simulink model "Simulink_Model"  (R2020b)
settings: Solver=FixedStepAuto  StartTime=0.0  StopTime=12  FixedStep=1  RelTol=1e-3
values from neighbouring files (symbols this model uses):
  ConstantA = Constants{1}    [Load_config.m]
  ConstantB = Constants{2}    [Load_config.m]
  ConstantC = Constants{3}    [Load_config.m]
  ConstantD = Constants{4}    [Load_config.m]
  ConstantE = Constants{5}    [Load_config.m]
  ConstantF = Constants{6}    [Load_config.m]
  ConstantG = Constants{7}    [Load_config.m]
  ConstantH = Constants{8}    [Load_config.m]
  ConstantI = Constants{9}    [Load_config.m]
  ConstantJ = Constants{18}    [Load_config.m]
  ConstantK = Constants{19}    [Load_config.m]
  ConstantL = Constants{20}    [Load_config.m]
  ConstantM = Constants{21}    [Load_config.m]
  ConstantO = Constants{22}    [Load_config.m]
undefined symbols (not defined in the file or in its folder): A1052, A2, F2, G1052, H2, K1052
libraries: simulink x32, sldvlib x22
(part 1 of 3)
settings Model: Creator=Marcus  LastModifiedBy=marcushanikat
settings ConfigComp: DVMode=PropertyProving  DVMaxProcessTime=36000  DVParameters=on  DVParametersUseConfig=on  DVTestConditions=EnableAll  DVTestObjectives=EnableAll  DVMaxTestCaseSteps=1000  DVTestSuiteOptimization=LongTestcases  DVDetectOutOfBounds=on  DVMaxViolationSteps=8

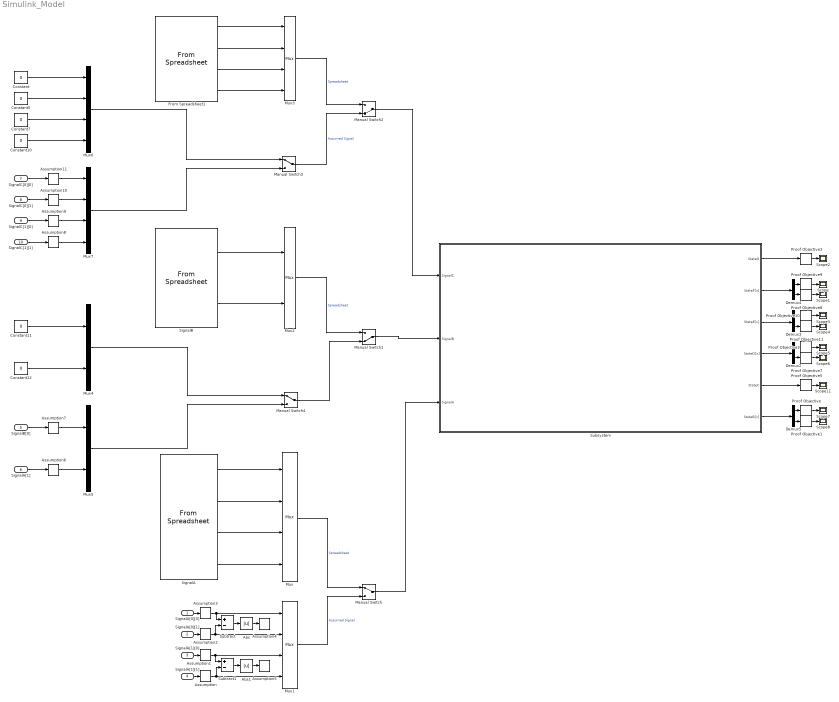
== system Simulink_Model ==
  SignalA[0][0] : Inport  OutDataTypeStr=int32
  SignalA[0][1] : Inport  Port=2  OutDataTypeStr=int32
  SignalA[1][0] : Inport  Port=3  OutDataTypeStr=int32
  SignalA[1][1] : Inport  Port=4  OutDataTypeStr=int32
  SignalB[0] : Inport  Port=5
  SignalA[1] : Inport  Port=6
  SignalC[0][0] : Inport  Port=7
  SignalC[0][1] : Inport  Port=8
  SignalC[1][0] : Inport  Port=9
  SignalC[1][1] : Inport  Port=10
  Abs : Abs
  Abs1 : Abs
  Assumption{,1..3} (4 alike) : sldvlib/Objectives and Constraints/Assumption  enabled=on  customAVTBlockType=Assumption  intervals={0 1 2 3 4 5}  initial=off  dispValues=off  outEnabled=on
      settings: SourceProductBaseCode=SL
  Assumption{8..11} (4 alike) : sldvlib/Objectives and Constraints/Assumption  enabled=on  customAVTBlockType=Assumption  intervals={0 1}  initial=off  dispValues=off  outEnabled=on
      settings: SourceProductBaseCode=SL
  Assumption4 : sldvlib/Objectives and Constraints/Assumption  enabled=on  customAVTBlockType=Assumption  intervals={0 1}  initial=off  dispValues=off  outEnabled=off
      settings: SourceProductBaseCode=SL
  Assumption5 : sldvlib/Objectives and Constraints/Assumption  enabled=on  customAVTBlockType=Assumption  intervals={0 1}  initial=off  dispValues=off  outEnabled=off
      settings: SourceProductBaseCode=SL
  Assumption6 : sldvlib/Objectives and Constraints/Assumption  enabled=on  customAVTBlockType=Assumption  intervals={0 1 2}  initial=off  dispValues=off  outEnabled=on
      settings: SourceProductBaseCode=SL
  Assumption7 : sldvlib/Objectives and Constraints/Assumption  enabled=on  customAVTBlockType=Assumption  intervals={0 1 2}  initial=off  dispValues=off  outEnabled=on
      settings: SourceProductBaseCode=SL
  Constant{,5,7,10..12} (6 alike) : Constant  Value=0
  Demux{2..5} (4 alike) : Demux  Outputs=2
  From Spreadsheet1 : FromSpreadsheet  FileName=/Users/marcushanikat/Documents/git/Master_thesis/Excel/Signals.xlsx  SheetName=Signals  Range=A2:A1052,H2:K1052  OutDataTypeStr=int32
  Manual Switch : ManualSwitch
  Manual Switch1 : ManualSwitch  CurrentSetting=0
  Manual Switch2 : ManualSwitch  CurrentSetting=0
  Manual Switch3 : ManualSwitch
  Manual Switch4 : ManualSwitch
  Mux{,1,3,6..7} (5 alike) : Mux
  Mux2 : Mux  Inputs=2
  Mux4 : Mux  Inputs=2
  Mux5 : Mux  Inputs=2
  Proof Objective{,1..3,5,7..11} (10 alike) : sldvlib/Objectives and Constraints/Proof Objective  enabled=off  customAVTBlockType=Proof Objective  intervals={0}  dispValues=off  outEnabled=on  enableStopSim=off
      settings: SourceProductBaseCode=SL
  Scope{,1..8,11} (10 alike) : Scope
  SignalA : FromSpreadsheet  FileName=/Users/marcushanikat/Documents/git/Master_thesis/Excel/Signals.xlsx  SheetName=Signals  Range=A2:E1052  OutDataTypeStr=int32
  SignalB : FromSpreadsheet  FileName=/Users/marcushanikat/Documents/git/Master_thesis/Excel/Signals.xlsx  SheetName=Signals  Range=A2:A1052,F2:G1052  OutDataTypeStr=int32
  Subsystem : Subsystem
  Subtract : Sum  Inputs=+-
  Subtract1 : Sum  Inputs=+-
  wires:
  SignalA[1][0]/1 -> Assumption1/1
  SignalA[1][1]/1 -> Assumption/1
  Assumption/1 -> Subtract1/2, Mux1/4
  SignalA/3 -> Mux/3
  SignalA/4 -> Mux/4
  SignalA/1 -> Mux/1
  SignalA/2 -> Mux/2
  Assumption1/1 -> Subtract1/1, Mux1/3
  Manual Switch/1 -> Subsystem/3(SignalA)
  Mux1/1 -> Manual Switch/2  "Assumed Signal"
  Mux/1 -> Manual Switch/1  "Spreadsheet"
  SignalB/2 -> Mux2/2
  SignalB/1 -> Mux2/1
  From Spreadsheet1/1 -> Mux3/1
  From Spreadsheet1/2 -> Mux3/2
  From Spreadsheet1/3 -> Mux3/3
  From Spreadsheet1/4 -> Mux3/4
  SignalA[1]/1 -> Assumption6/1
  SignalB[0]/1 -> Assumption7/1
  SignalC[1][1]/1 -> Assumption8/1
  SignalC[0][1]/1 -> Assumption10/1
  SignalC[0][0]/1 -> Assumption11/1
  SignalC[1][0]/1 -> Assumption9/1
  Manual Switch1/1 -> Subsystem/2(SignalB)
  Mux2/1 -> Manual Switch1/1  "Spreadsheet"
  Manual Switch2/1 -> Subsystem/1(SignalC)
  Manual Switch3/1 -> Manual Switch2/2  "Assumed Signal"
  Mux3/1 -> Manual Switch2/1  "Spreadsheet"
  Subsystem/6(StateB[x]) -> Demux5/1
  Subsystem/3(StateE[x]) -> Demux3/1
  Subsystem/2(StateF[x]) -> Demux4/1
  Subsystem/4(StateD[x]) -> Demux2/1
  Subsystem/5(StateC) -> Proof Objective5/1
  Demux5/1 -> Proof Objective/1
  Proof Objective/1 -> Scope7/1
  Demux5/2 -> Proof Objective1/1
  Proof Objective1/1 -> Scope8/1
  Demux2/1 -> Proof Objective2/1
  Proof Objective2/1 -> Scope5/1
  Proof Objective3/1 -> Scope2/1
  Subsystem/1(StateG) -> Proof Objective3/1
  Proof Objective5/1 -> Scope11/1
  Subtract/1 -> Abs/1
  Assumption3/1 -> Subtract/1, Mux1/1
  Assumption2/1 -> Subtract/2, Mux1/2
  SignalA[0][1]/1 -> Assumption2/1
  SignalA[0][0]/1 -> Assumption3/1
  Abs/1 -> Assumption4/1
  Subtract1/1 -> Abs1/1
  Abs1/1 -> Assumption5/1
  Constant10/1 -> Mux6/4
  Constant7/1 -> Mux6/3
  Constant5/1 -> Mux6/2
  Constant/1 -> Mux6/1
  Assumption11/1 -> Mux7/1
  Assumption10/1 -> Mux7/2
  Assumption9/1 -> Mux7/3
  Assumption8/1 -> Mux7/4
  Mux7/1 -> Manual Switch3/2
  Mux6/1 -> Manual Switch3/1
  Constant11/1 -> Mux4/1
  Constant12/1 -> Mux4/2
  Assumption7/1 -> Mux5/1
  Assumption6/1 -> Mux5/2
  Manual Switch4/1 -> Manual Switch1/2
  Mux5/1 -> Manual Switch4/2
  Mux4/1 -> Manual Switch4/1
  Demux2/2 -> Proof Objective7/1
  Proof Objective7/1 -> Scope6/1
  Demux4/2 -> Proof Objective8/1
  Proof Objective8/1 -> Scope1/1
  Demux4/1 -> Proof Objective9/1
  Proof Objective9/1 -> Scope/1
  Demux3/1 -> Proof Objective10/1
  Proof Objective10/1 -> Scope3/1
  Demux3/2 -> Proof Objective11/1
  Proof Objective11/1 -> Scope4/1

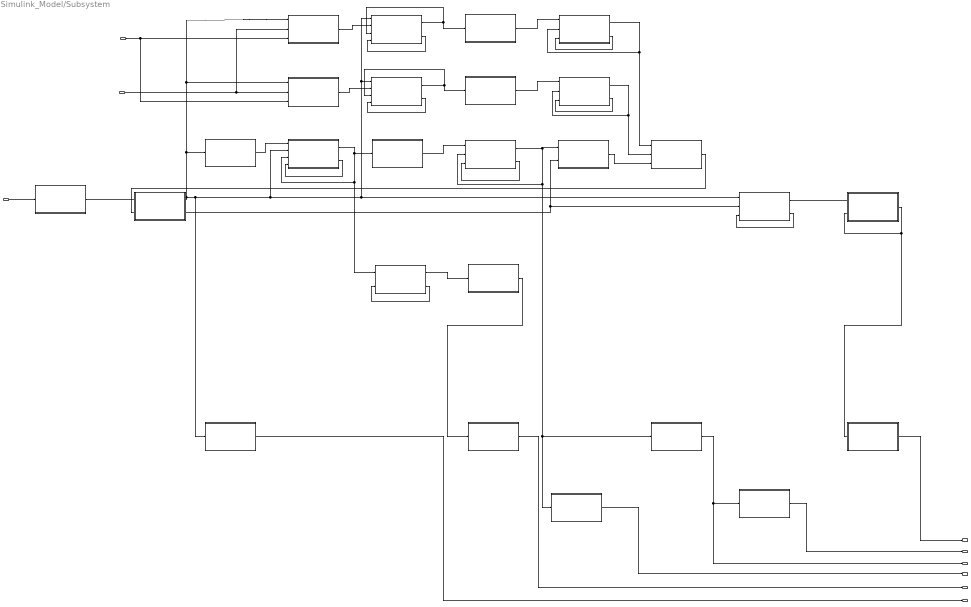
== system Simulink_Model/Subsystem ==
  SignalC : Inport
  SignalB : Inport  Port=2
  SignalA : Inport  Port=3
  Requirement1 : Subsystem  TreatAsAtomicUnit=on
  Requirement10 : Subsystem  TreatAsAtomicUnit=on
  Requirement11 : Subsystem  TreatAsAtomicUnit=on
  Requirement12 : Subsystem  TreatAsAtomicUnit=on
  Requirement14 : Subsystem  TreatAsAtomicUnit=on
  Requirement15 : Subsystem  TreatAsAtomicUnit=on
  Requirement2 : Subsystem  TreatAsAtomicUnit=on
  Requirement20 : Subsystem  TreatAsAtomicUnit=on
  Requirement21 : Subsystem  TreatAsAtomicUnit=on
  Requirement23 : Subsystem  TreatAsAtomicUnit=on
  Requirement24 : Subsystem  TreatAsAtomicUnit=on
  Requirement25 : Subsystem  TreatAsAtomicUnit=on
  Requirement26 : Subsystem  TreatAsAtomicUnit=on
  Requirement3 : Subsystem  TreatAsAtomicUnit=on
  Requirement4 : Subsystem  TreatAsAtomicUnit=on
  Requirement5 : Subsystem  TreatAsAtomicUnit=on
  Requirement6 : Subsystem  TreatAsAtomicUnit=on
  Requirement7 : Subsystem  TreatAsAtomicUnit=on
  Requirement8 : Subsystem  TreatAsAtomicUnit=on
  Requirement9 : Subsystem  TreatAsAtomicUnit=on
  Verification2 : Subsystem  TreatAsAtomicUnit=on
  Verification3 : Subsystem  TreatAsAtomicUnit=on
  Verification4 : Subsystem  TreatAsAtomicUnit=on
  Verification5 : Subsystem  TreatAsAtomicUnit=on
  Verification6 : Subsystem  TreatAsAtomicUnit=on
  Verification8 : Subsystem  TreatAsAtomicUnit=on
  StateG : Outport
  StateF[x] : Outport  Port=2
  StateE[x] : Outport  Port=3
  StateD[x] : Outport  Port=4
  StateC : Outport  Port=5
  StateB[x] : Outport  Port=6
  wires:
  Requirement7/1(OutputJ) -> Requirement8/2(OutputJ)  "OutputJ"
  Requirement2/2(OutputC) -> Requirement20/2(OutputC), Requirement25/2(OutputC)  "OutputC"
  Requirement14/2(OutputS) -> Requirement14/3(OutputSOld)
  Requirement15/1(OutputT) -> Requirement21/1(OutputT), Requirement15/2(OutputTOld)  "OutputT"
  Requirement20/1(OutputV) -> Requirement21/3(OutputV)  "OutputV"
  Requirement2/1(OutputB) -> Verification2/1(OutputB), Requirement4/2(OutputB), Requirement25/1(OutputB), Requirement8/1(OutputB), Requirement6/1(OutputB), Requirement7/1(OutputB), Requirement5/1(OutputB), Requirement3/1(OutputB)  "OutputB"
  Requirement4/1(OutputE) -> Requirement4/3(OutputEOld), Requirement23/1(OutputE), Requirement9/1(OutputE)  "OutputE"
  Requirement12/1(OutputP) -> Requirement12/2(OutputPOld), Verification5/1(OutputP), Verification4/1(OutputP), Requirement20/1(OutputP)  "OutputP"
  Requirement10/1(OutputN) -> Requirement14/1(OutputN)  "OutputN"
  Requirement14/1(OutputR) -> Requirement14/2(OutputROld), Requirement21/2(OutputR)  "OutputR"
  Requirement21/1(OutputW) -> Requirement2/2(OutputW)
  Requirement24/1(OutputY) -> Verification3/1(OutputY)  "OutputY"
  Requirement15/2(OutputU) -> Requirement15/3(OutputUOld)
  Requirement11/1(OutputO) -> Requirement15/1(OutputO)  "OutputO"
  Verification8/1(StateG) -> StateG/1  "StateG"
  Verification3/1(StateC) -> StateC/1  "StateC"
  Requirement4/2(OutputF) -> Requirement4/4(OutputFOld)
  Verification5/1(StateE) -> Verification6/1(StateE), StateE[x]/1  "StateE"
  Requirement5/1(OutputG) -> Requirement6/2(OutputG)  "OutputG"
  Verification4/1(StateD) -> StateD[x]/1  "StateD"
  Requirement25/2(OutputAA) -> Requirement25/3(OutputAAOld)
  Requirement3/1(OutputD) -> Requirement4/1(OutputD)  "OutputD"
  Requirement25/1(OutputZ) -> Requirement26/1(OutputZ)  "OutputZ"
  Verification2/1(StateB) -> StateB[x]/1  "StateB"
  Requirement8/1(OutputK) -> Requirement11/1(OutputK), Requirement8/3(OutputKOld)  "OutputK"
  Verification6/1(StateF) -> StateF[x]/1  "StateF"
  Requirement6/1(OutputH) -> Requirement6/3(OutputHOld), Requirement10/1(OutputH)  "OutputH"
  Requirement8/2(OutputL) -> Requirement8/4(OutputLOld)
  Requirement23/2(OutputE(t-2)) -> Requirement23/2(OutputEOld)
  Requirement23/1(OutputX) -> Requirement24/1(OutputX)  "OutputX"
  SignalA/1 -> Requirement1/1(SignalA)
  Requirement1/1(OutputA) -> Requirement2/1(OutputA)
  Requirement12/2(OutputQ) -> Requirement12/3(OutputQOld)
  Requirement9/1(OutputM) -> Requirement12/1(OutputM)
  Requirement6/2(OutputI) -> Requirement6/4(OutputIOld)
  Requirement26/1(OutputAB) -> Verification8/1(OutputAB), Requirement26/2(OutputABOld)  "OutputAB"
  SignalC/1 -> Requirement5/3(SignalC), Requirement7/3(SignalC)
  SignalB/1 -> Requirement7/2(SignalB), Requirement5/2(SignalB)

== system Simulink_Model/Subsystem/Requirement1 ==
  note: Requirements implemented:
      | Requirement1
  SignalA : Inport
  Compare To Constant : simulink/Logic and Bit Operations/Compare To Constant  relop===  const=2  OutDataTypeStr=boolean
  Compare To Constant1 : simulink/Logic and Bit Operations/Compare To Constant  relop===  const=2  OutDataTypeStr=boolean
  Constant : Constant  Value=ConstantA
  Constant1 : Constant  Value=ConstantA
  Demux : Demux
  Gain{,1..3} (4 alike) : Gain  Gain=-1
  Mux : Mux
  Switch{,1..3} (4 alike) : Switch  Criteria=u2 > Threshold  OutDataTypeStr=int32
  OutputA : Outport
  wires:
  SignalA/1 -> Demux/1
  Constant1/1 -> Compare To Constant/1  "ConstantA"
  Compare To Constant/1 -> Switch1/2, Switch/2
  Demux/1 -> Gain/1, Switch/3
  Switch/1 -> Mux/1
  Gain/1 -> Switch/1
  Switch1/1 -> Mux/2
  Demux/2 -> Gain1/1, Switch1/3
  Gain1/1 -> Switch1/1
  Constant/1 -> Compare To Constant1/1  "ConstantA"
  Switch2/1 -> Mux/3
  Demux/3 -> Gain2/1, Switch2/3
  Gain2/1 -> Switch2/1
  Switch3/1 -> Mux/4
  Demux/4 -> Switch3/3, Gain3/1
  Gain3/1 -> Switch3/1
  Compare To Constant1/1 -> Switch2/2, Switch3/2
  Mux/1 -> OutputA/1

== system Simulink_Model/Subsystem/Requirement10 ==
  note: Requirements implemented:
      | Requirement10
  OutputH : Inport
  Demux : Demux
  Max : MinMax  Function=max  Inputs=2
  Max1 : MinMax  Function=max  Inputs=2
  Mux : Mux  Inputs=2
  OutputN : Outport
  wires:
  OutputH/1 -> Demux/1
  Mux/1 -> OutputN/1
  Demux/2 -> Max/2
  Demux/1 -> Max/1
  Demux/3 -> Max1/1
  Demux/4 -> Max1/2
  Max1/1 -> Mux/2
  Max/1 -> Mux/1

== system Simulink_Model/Subsystem/Requirement11 ==
  note: Requirements implemented:
      | Requirement11
  OutputK : Inport
  Demux : Demux
  Min : MinMax  Inputs=2
  Min1 : MinMax  Inputs=2
  Mux : Mux  Inputs=2
  OutputO : Outport
  wires:
  OutputK/1 -> Demux/1
  Mux/1 -> OutputO/1
  Demux/1 -> Min/1
  Demux/2 -> Min/2
  Demux/3 -> Min1/1
  Demux/4 -> Min1/2
  Min/1 -> Mux/1
  Min1/1 -> Mux/2

== system Simulink_Model/Subsystem/Requirement12 ==
  note: Requirements implemented:
      | Requirement12
  OutputM : Inport
  OutputPOld : Inport  Port=2
  OutputQOld : Inport  Port=3
  ComputeOutput0 : Subsystem
  ComputeOutput1 : Subsystem
  Demux : Demux  Outputs=2
  Demux1 : Demux  Outputs=2
  Demux2 : Demux  Outputs=2
  Mux : Mux  Inputs=2
  Mux1 : Mux  Inputs=2
  OutputP : Outport
  OutputQ : Outport  Port=2
  wires:
  OutputPOld/1 -> Demux1/1
  OutputM/1 -> Demux/1
  OutputQOld/1 -> Demux2/1
  Mux1/1 -> OutputQ/1
  Mux/1 -> OutputP/1
  ComputeOutput1/1(OutputP[x]) -> Mux/2
  ComputeOutput0/1(OutputP[x]) -> Mux/1
  ComputeOutput0/2(OutputQ[x]) -> Mux1/1
  ComputeOutput1/2(OutputQ[x]) -> Mux1/2
  Demux/1 -> ComputeOutput0/1(OutputM[x])
  Demux/2 -> ComputeOutput1/1(OutputM[x])
  Demux1/1 -> ComputeOutput0/2(OutputPOld[x])
  Demux1/2 -> ComputeOutput1/2(OutputPOld[x])
  Demux2/1 -> ComputeOutput0/3(OutputQOld[x])
  Demux2/2 -> ComputeOutput1/3(OutputQOld[x])

== system Simulink_Model/Subsystem/Requirement14 ==
  note: Requirements implemented:
      | Requirement14
  OutputN : Inport
  OutputROld : Inport  Port=2
  OutputSOld : Inport  Port=3
  ComputeOutput0 : Subsystem
  ComputeOutput1 : Subsystem
  Demux : Demux  Outputs=2
  Demux1 : Demux  Outputs=2
  Demux2 : Demux  Outputs=2
  Mux : Mux  Inputs=2
  Mux1 : Mux  Inputs=2
  OutputR : Outport
  OutputS : Outport  Port=2
  wires:
  Mux/1 -> OutputS/1
  Mux1/1 -> OutputR/1
  ComputeOutput0/1(OutputR[x]) -> Mux1/1
  ComputeOutput1/1(OutputR[x]) -> Mux1/2
  ComputeOutput0/2(OutputS[x]) -> Mux/1
  ComputeOutput1/2(OutputS[x]) -> Mux/2
  OutputN/1 -> Demux/1
  OutputROld/1 -> Demux1/1
  OutputSOld/1 -> Demux2/1
  Demux/1 -> ComputeOutput0/1(OutputN[x])
  Demux/2 -> ComputeOutput1/1(OutputN[x])
  Demux1/1 -> ComputeOutput0/2(OutputROld[x])
  Demux1/2 -> ComputeOutput1/2(OutputROld[x])
  Demux2/1 -> ComputeOutput0/3(OutputSOld[x])
  Demux2/2 -> ComputeOutput1/3(OutputSOld[x])

== system Simulink_Model/Subsystem/Requirement15 ==
  note: Requirements implemented:
      | Requirement15
  OutputO : Inport
  OutputTOld : Inport  Port=2
  OutputUOld : Inport  Port=3
  ComputeOutput0 : Subsystem
  ComputeOutput1 : Subsystem
  Demux : Demux  Outputs=2
  Demux1 : Demux  Outputs=2
  Demux2 : Demux  Outputs=2
  Mux : Mux  Inputs=2
  Mux1 : Mux  Inputs=2
  OutputT : Outport
  OutputU : Outport  Port=2
  wires:
  Mux1/1 -> OutputU/1
  ComputeOutput1/2(OutputU[x]) -> Mux1/2
  ComputeOutput1/1(OutputT[x]) -> Mux/2
  Mux/1 -> OutputT/1
  ComputeOutput0/1(OutputT[x]) -> Mux/1
  ComputeOutput0/2(OutputU[x]) -> Mux1/1
  OutputTOld/1 -> Demux1/1
  OutputO/1 -> Demux/1
  OutputUOld/1 -> Demux2/1
  Demux/1 -> ComputeOutput0/1(OutputO[x])
  Demux/2 -> ComputeOutput1/1(OutputO[x])
  Demux1/1 -> ComputeOutput0/2(OutputTOld[x])
  Demux1/2 -> ComputeOutput1/2(OutputTOld[x])
  Demux2/1 -> ComputeOutput0/3(OutputUOld[x])
  Demux2/2 -> ComputeOutput1/3(OutputUOld[x])

== system Simulink_Model/Subsystem/Requirement2 ==
  note: Requirements implemented:
      | Requirement2
  OutputA : Inport
  OutputW : Inport  Port=2
  Add : Sum
  Add1 : Sum
  Constant : Constant  Value=0
  Constant1 : Constant
  Constant2 : Constant  Value=-1
  Delay : Delay  DelayLength=1  InitialCondition=0
  Delay1 : Delay  DelayLength=1  InitialCondition=0
  Demux : Demux
  Demux1 : Demux  Outputs=2
  Gain{,1..3} (4 alike) : Gain  Gain=-1
  Mux : Mux  Inputs=2
  Mux1 : Mux
  Product : Product  OutDataTypeStr=int32
  Product1 : Product  OutDataTypeStr=int32
  Relational Operator : RelationalOperator  Operator=>  OutDataTypeStr=boolean  RndMeth=Simplest
  Relational Operator1 : RelationalOperator  Operator=>  OutDataTypeStr=boolean  RndMeth=Simplest
  Switch{,1..3} (4 alike) : Switch  Criteria=u2 > Threshold  OutDataTypeStr=int32
  Switch4 : Switch  Criteria=u2 > Threshold
  Switch5 : Switch  Criteria=u2 > Threshold
  OutputB : Outport
  OutputC : Outport  Port=2
  wires:
  OutputA/1 -> Demux/1
  Demux/1 -> Gain/1, Switch/1, Add/1
  Demux/2 -> Gain1/1, Switch1/1, Add/2
  Demux/4 -> Switch3/1, Gain3/1, Add1/2
  Demux/3 -> Switch2/1, Gain2/1, Add1/1
  Add/1 -> Product/1
  Add1/1 -> Product1/1
  OutputW/1 -> Demux1/1
  Demux1/1 -> Delay/1
  Product/1 -> Relational Operator/1
  Demux1/2 -> Delay1/1
  Constant/1 -> Relational Operator/2, Relational Operator1/2
  Product1/1 -> Relational Operator1/1
  Relational Operator/1 -> Switch4/2, Switch1/2, Switch/2
  Relational Operator1/1 -> Switch5/2, Switch2/2, Switch3/2
  Mux/1 -> OutputC/1
  Switch/1 -> Mux1/1
  Switch1/1 -> Mux1/2
  Switch2/1 -> Mux1/3
  Switch3/1 -> Mux1/4
  Mux1/1 -> OutputB/1
  Gain/1 -> Switch/3
  Gain1/1 -> Switch1/3
  Gain2/1 -> Switch2/3
  Gain3/1 -> Switch3/3
  Delay/1 -> Product/2
  Switch4/1 -> Mux/1
  Switch5/1 -> Mux/2
  Constant2/1 -> Switch4/3, Switch5/3
  Constant1/1 -> Switch5/1, Switch4/1
  Delay1/1 -> Product1/2

== system Simulink_Model/Subsystem/Requirement20 ==
  note: Requirements implemented:
      | Requirement20
  OutputP : Inport
  OutputC : Inport  Port=2
  Compare To Constant : simulink/Logic and Bit Operations/Compare To Constant  relop=>  const=0  OutDataTypeStr=boolean
  Compare To Constant1 : simulink/Logic and Bit Operations/Compare To Constant  relop===  const=0  OutDataTypeStr=boolean
  Compare To Constant2 : simulink/Logic and Bit Operations/Compare To Constant  relop=>  const=0  OutDataTypeStr=boolean
  Compare To Constant3 : simulink/Logic and Bit Operations/Compare To Constant  relop===  const=0  OutDataTypeStr=boolean
  Constant : Constant
  Constant1 : Constant  Value=0
  Constant2 : Constant  Value=-1
  Constant3 : Constant
  Constant4 : Constant  Value=0
  Constant5 : Constant  Value=-1
  Demux : Demux  Outputs=2
  Demux1 : Demux  Outputs=2
  Mux : Mux  Inputs=2
  Product : Product
  Product1 : Product
  Switch{,1..3} (4 alike) : Switch  Criteria=u2 > Threshold
  OutputV : Outport
  wires:
  OutputP/1 -> Demux/1
  OutputC/1 -> Demux1/1
  Demux/1 -> Product/1
  Demux1/1 -> Product/2
  Demux1/2 -> Product1/2
  Demux/2 -> Product1/1
  Product/1 -> Compare To Constant1/1, Compare To Constant/1
  Compare To Constant/1 -> Switch/2
  Constant/1 -> Switch/1
  Compare To Constant1/1 -> Switch1/2
  Constant1/1 -> Switch1/1
  Constant2/1 -> Switch1/3
  Switch1/1 -> Switch/3
  Switch3/1 -> Switch2/3
  Constant4/1 -> Switch3/1
  Compare To Constant3/1 -> Switch3/2
  Compare To Constant2/1 -> Switch2/2
  Constant3/1 -> Switch2/1
  Constant5/1 -> Switch3/3
  Product1/1 -> Compare To Constant3/1, Compare To Constant2/1
  Mux/1 -> OutputV/1
  Switch/1 -> Mux/1
  Switch2/1 -> Mux/2

== system Simulink_Model/Subsystem/Requirement21 ==
  note: Requirements implemented:
      | Requirement21
  OutputT : Inport
  OutputR : Inport  Port=2
  OutputV : Inport  Port=3
  Compare To Constant : simulink/Logic and Bit Operations/Compare To Constant  relop=>  const=0  OutDataTypeStr=boolean
  Compare To Constant1 : simulink/Logic and Bit Operations/Compare To Constant  relop=>  const=0  OutDataTypeStr=boolean
  Constant : Constant  Value=0
  Demux1 : Demux  Outputs=2
  Demux2 : Demux  Outputs=2
  Demux3 : Demux  Outputs=2
  Mux : Mux  Inputs=2
  Product : Product
  Product1 : Product
  Switch : Switch  Criteria=u2 > Threshold
  Switch1 : Switch  Criteria=u2 > Threshold
  OutputW : Outport
  wires:
  OutputV/1 -> Demux2/1
  OutputR/1 -> Demux1/1
  Mux/1 -> OutputW/1
  OutputT/1 -> Demux3/1
  Demux3/1 -> Product/1
  Product/1 -> Compare To Constant/1
  Product1/1 -> Compare To Constant1/1
  Demux1/2 -> Product1/2
  Compare To Constant1/1 -> Switch/2
  Compare To Constant/1 -> Switch1/2
  Demux2/1 -> Switch1/1
  Demux2/2 -> Switch/1
  Constant/1 -> Switch1/3, Switch/3
  Switch1/1 -> Mux/1
  Switch/1 -> Mux/2
  Demux1/1 -> Product/2
  Demux3/2 -> Product1/1

== system Simulink_Model/Subsystem/Requirement23 ==
  note: Requirements implemented:
      | Requirement23
  OutputE : Inport
  OutputEOld : Inport  Port=2
  Delay{,1..3} (4 alike) : Delay  InitialCondition=0
  Demux : Demux
  Demux1 : Demux
  Mux : Mux
  OutputX[0][0] : Subsystem
  OutputX[0][1] : Subsystem
  OutputX[1][0] : Subsystem
  OutputX[1][1] : Subsystem
  OutputX : Outport
  OutputE(t-2) : Outport  Port=2
  wires:
  OutputE/1 -> Demux/1, OutputE(t-2)/1
  Demux/1 -> OutputX[0][0]/1(OutputE[x][y])
  Demux/3 -> OutputX[1][0]/1(OutputE[x][y])
  Demux/2 -> OutputX[0][1]/1(OutputE[x][y])
  Demux/4 -> OutputX[1][1]/1(OutputE[x][y])
  Demux1/1 -> Delay/1
  Demux1/2 -> Delay1/1
  Demux1/3 -> Delay2/1
  Demux1/4 -> Delay3/1
  Mux/1 -> OutputX/1
  OutputX[0][0]/1(OutputX[x][y]) -> Mux/1
  OutputX[0][1]/1(OutputX[x][y]) -> Mux/2
  OutputX[1][0]/1(OutputX[x][y]) -> Mux/3
  OutputX[1][1]/1(OutputX[x][y]) -> Mux/4
  OutputEOld/1 -> Demux1/1
  Delay/1 -> OutputX[0][0]/2(OutputEOld[x][y])
  Delay1/1 -> OutputX[0][1]/2(OutputEOld[x][y])
  Delay2/1 -> OutputX[1][0]/2(OutputEOld[x][y])
  Delay3/1 -> OutputX[1][1]/2(OutputEOld[x][y])

== system Simulink_Model/Subsystem/Requirement24 ==
  note: Requirements implemented:
      | Requirement24
  OutputX : Inport
  Demux : Demux
  Mux : Mux  Inputs=2
  OutputY[0] : Subsystem
  OutputY[1] : Subsystem
  OutputY : Outport
  wires:
  OutputX/1 -> Demux/1
  Demux/4 -> OutputY[1]/2(OutputX[x][1])
  Demux/3 -> OutputY[1]/1(OutputX[x][0])
  Demux/2 -> OutputY[0]/2(OutputX[x][1])
  Demux/1 -> OutputY[0]/1(OutputX[x][0])
  Mux/1 -> OutputY/1
  OutputY[0]/1(OutputY[x]) -> Mux/1
  OutputY[1]/1(OutputY[x]) -> Mux/2

== system Simulink_Model/Subsystem/Requirement25 ==
  note: Requirements implemented:
      | Requirement25
  OutputB : Inport
  OutputC : Inport  Port=2
  OutputAAOld : Inport  Port=3
  Delay : Delay  DelayLength=1  InitialCondition=0
  Delay1 : Delay  DelayLength=1  InitialCondition=0
  Demux : Demux
  Demux1 : Demux  Outputs=2
  Demux2 : Demux  Outputs=2
  Mux : Mux  Inputs=2
  Mux1 : Mux  Inputs=2
  Subsystem : Subsystem
  Subsystem1 : Subsystem
  Terminator : Terminator
  Terminator1 : Terminator
  OutputZ : Outport
  OutputAA : Outport  Port=2
  wires:
  Mux/1 -> OutputZ/1
  Mux1/1 -> OutputAA/1
  OutputAAOld/1 -> Demux2/1
  OutputC/1 -> Demux1/1
  OutputB/1 -> Demux/1
  Demux2/1 -> Delay/1
  Demux2/2 -> Delay1/1
  Subsystem/1(OutputZ[x]) -> Mux/1
  Subsystem1/1(OutputZ[x]) -> Mux/2
  Subsystem/2(OutputAA[x]) -> Mux1/1
  Subsystem1/2(OutputAA[x]) -> Mux1/2
  Demux/1 -> Subsystem/1(OutputB[x][0])
  Demux/3 -> Subsystem1/1(OutputB[x][0])
  Demux1/1 -> Subsystem/2(OutputC[x])
  Demux1/2 -> Subsystem1/2(OutputC[x])
  Delay/1 -> Subsystem/3(OutputAAOld[x])
  Delay1/1 -> Subsystem1/3(OutputAAOld[x])
  Demux/2 -> Terminator/1
  Demux/4 -> Terminator1/1

== system Simulink_Model/Subsystem/Requirement26 ==
  note: Requirements implemented:
      | Requirement26
  OutputZ : Inport
  OutputABOld : Inport  Port=2
  Delay : Delay  DelayLength=1  InitialCondition=0
  Delay1 : Delay  DelayLength=1  InitialCondition=0
  Demux : Demux  Outputs=2
  Demux1 : Demux  Outputs=2
  Mux : Mux  Inputs=2
  Subsystem : Subsystem
  Subsystem1 : Subsystem
  OutputAB : Outport
  wires:
  OutputZ/1 -> Demux/1
  OutputABOld/1 -> Demux1/1
  Demux1/2 -> Delay1/1
  Demux1/1 -> Delay/1
  Mux/1 -> OutputAB/1
  Subsystem/1(OutputAB[x]) -> Mux/1
  Subsystem1/1(OutputAB[x]) -> Mux/2
  Demux/1 -> Subsystem/1(OutputZ[x])
  Demux/2 -> Subsystem1/1(OutputZ[x])
  Delay/1 -> Subsystem/2(OutputABOld[x])
  Delay1/1 -> Subsystem1/2(OutputABOld[x])

== system Simulink_Model/Subsystem/Requirement3 ==
  note: Requirements implemented:
      | Requirement3
  OutputB : Inport
  ComputeOutputD[0][0] : Subsystem
  ComputeOutputD[0][1] : Subsystem
  ComputeOutputD[1][0] : Subsystem
  ComputeOutputD[1][1] : Subsystem
  Demux : Demux
  Mux : Mux
  OutputD : Outport
  wires:
  OutputB/1 -> Demux/1
  Demux/4 -> ComputeOutputD[1][1]/1(OutputB[x][y])
  Demux/3 -> ComputeOutputD[1][0]/1(OutputB[x][y])
  Demux/2 -> ComputeOutputD[0][1]/1(OutputB[x][y])
  Demux/1 -> ComputeOutputD[0][0]/1(OutputB[x][y])
  ComputeOutputD[0][0]/1(OutputD[x][y]) -> Mux/1
  ComputeOutputD[0][1]/1(OutputD[x][y]) -> Mux/2
  ComputeOutputD[1][0]/1(OutputD[x][y]) -> Mux/3
  ComputeOutputD[1][1]/1(OutputD[x][y]) -> Mux/4
  Mux/1 -> OutputD/1

== system Simulink_Model/Subsystem/Requirement4 ==
  note: Requirements implemented:
      | Requirement4
  OutputD : Inport
  OutputB : Inport  Port=2
  OutputEOld : Inport  Port=3
  OutputFOld : Inport  Port=4
  ComputeOutput[0][0] : Subsystem
  ComputeOutput[0][1] : Subsystem
  ComputeOutput[1][0] : Subsystem
  ComputeOutput[1][1] : Subsystem
  Demux{,1..3} (4 alike) : Demux
  Mux : Mux
  Mux1 : Mux
  OutputE : Outport
  OutputF : Outport  Port=2
  wires:
  OutputFOld/1 -> Demux3/1
  OutputEOld/1 -> Demux2/1
  OutputB/1 -> Demux1/1
  OutputD/1 -> Demux/1
  Demux/1 -> ComputeOutput[0][0]/2(OutputD[x][y])
  Demux1/1 -> ComputeOutput[0][0]/1(OutputB[x][y])
  Demux2/1 -> ComputeOutput[0][0]/3(OutputEOld[x][y])
  Demux3/1 -> ComputeOutput[0][0]/4(OutputFOld[x][y])
  Mux/1 -> OutputE/1
  ComputeOutput[0][0]/1(OutputE[x][y]) -> Mux/1
  Mux1/1 -> OutputF/1
  ComputeOutput[0][0]/2(OutputF[x][y]) -> Mux1/1
  Demux3/4 -> ComputeOutput[1][1]/4(OutputFOld[x][y])
  Demux3/3 -> ComputeOutput[1][0]/4(OutputFOld[x][y])
  Demux3/2 -> ComputeOutput[0][1]/4(OutputFOld[x][y])
  Demux2/2 -> ComputeOutput[0][1]/3(OutputEOld[x][y])
  Demux2/3 -> ComputeOutput[1][0]/3(OutputEOld[x][y])
  Demux2/4 -> ComputeOutput[1][1]/3(OutputEOld[x][y])
  Demux/2 -> ComputeOutput[0][1]/2(OutputD[x][y])
  Demux/3 -> ComputeOutput[1][0]/2(OutputD[x][y])
  Demux/4 -> ComputeOutput[1][1]/2(OutputD[x][y])
  Demux1/2 -> ComputeOutput[0][1]/1(OutputB[x][y])
  Demux1/3 -> ComputeOutput[1][0]/1(OutputB[x][y])
  Demux1/4 -> ComputeOutput[1][1]/1(OutputB[x][y])
  ComputeOutput[0][1]/1(OutputE[x][y]) -> Mux/2
  ComputeOutput[1][0]/1(OutputE[x][y]) -> Mux/3
  ComputeOutput[1][1]/1(OutputE[x][y]) -> Mux/4
  ComputeOutput[1][1]/2(OutputF[x][y]) -> Mux1/4
  ComputeOutput[1][0]/2(OutputF[x][y]) -> Mux1/3
  ComputeOutput[0][1]/2(OutputF[x][y]) -> Mux1/2

== system Simulink_Model/Subsystem/Requirement5 ==
  note: Requirements implemented:
      | Requirement5
  OutputB : Inport
  SignalB : Inport  Port=2
  SignalC : Inport  Port=3
  ComputeOutputG[0][0] : Subsystem
  ComputeOutputG[0][1] : Subsystem
  ComputeOutputG[1][0] : Subsystem
  ComputeOutputG[1][1] : Subsystem
  Demux : Demux  Outputs=2
  Demux1 : Demux
  Demux2 : Demux
  Mux : Mux
  Scope : Scope
  OutputG : Outport
  wires:
  OutputB/1 -> Demux1/1
  SignalC/1 -> Demux2/1
  SignalB/1 -> Demux/1
  Mux/1 -> OutputG/1
  ComputeOutputG[0][0]/1(OutputG[x][y]) -> Mux/1, Scope/1
  ComputeOutputG[0][1]/1(OutputG[x][y]) -> Mux/2
  ComputeOutputG[1][0]/1(OutputG[x][y]) -> Mux/3
  ComputeOutputG[1][1]/1(OutputG[x][y]) -> Mux/4
  Demux1/1 -> ComputeOutputG[0][0]/1(OutputB[x][y])
  Demux1/2 -> ComputeOutputG[0][1]/1(OutputB[x][y])
  Demux1/3 -> ComputeOutputG[1][0]/1(OutputB[x][y])
  Demux1/4 -> ComputeOutputG[1][1]/1(OutputB[x][y])
  Demux/1 -> ComputeOutputG[0][1]/2(SignalB[x]), ComputeOutputG[0][0]/2(SignalB[x])
  Demux/2 -> ComputeOutputG[1][1]/2(SignalB[x]), ComputeOutputG[1][0]/2(SignalB[x])
  Demux2/1 -> ComputeOutputG[0][0]/3(SignalC[x][y])
  Demux2/2 -> ComputeOutputG[0][1]/3(SignalC[x][y])
  Demux2/3 -> ComputeOutputG[1][0]/3(SignalC[x][y])
  Demux2/4 -> ComputeOutputG[1][1]/3(SignalC[x][y])

== system Simulink_Model/Subsystem/Requirement6 ==
  note: Requirements implemented:
      | Requirement6
  OutputB : Inport
  OutputG : Inport  Port=2
  OutputHOld : Inport  Port=3
  OutputIOld : Inport  Port=4
  ComputeOutput[0][0] : Subsystem
  ComputeOutput[0][1] : Subsystem
  ComputeOutput[1][0] : Subsystem
  ComputeOutput[1][1] : Subsystem
  Demux{,1..3} (4 alike) : Demux
  Mux : Mux
  Mux1 : Mux
  OutputH : Outport
  OutputI : Outport  Port=2
  wires:
  OutputB/1 -> Demux/1
  OutputG/1 -> Demux1/1
  OutputHOld/1 -> Demux2/1
  OutputIOld/1 -> Demux3/1
  Demux/1 -> ComputeOutput[0][0]/1(OutputB[x][y])
  Demux1/1 -> ComputeOutput[0][0]/2(OutputG[x][y])
  Demux2/1 -> ComputeOutput[0][0]/3(OutputHOld[x][y])
  Demux3/1 -> ComputeOutput[0][0]/4(OutputIOld[x][y])
  Demux1/2 -> ComputeOutput[0][1]/2(OutputG[x][y])
  Demux/2 -> ComputeOutput[0][1]/1(OutputB[x][y])
  Demux2/2 -> ComputeOutput[0][1]/3(OutputHOld[x][y])
  Demux3/2 -> ComputeOutput[0][1]/4(OutputIOld[x][y])
  Demux2/3 -> ComputeOutput[1][0]/3(OutputHOld[x][y])
  Demux1/3 -> ComputeOutput[1][0]/2(OutputG[x][y])
  Demux/3 -> ComputeOutput[1][0]/1(OutputB[x][y])
  Demux3/3 -> ComputeOutput[1][0]/4(OutputIOld[x][y])
  Demux3/4 -> ComputeOutput[1][1]/4(OutputIOld[x][y])
  Demux2/4 -> ComputeOutput[1][1]/3(OutputHOld[x][y])
  Demux1/4 -> ComputeOutput[1][1]/2(OutputG[x][y])
  Demux/4 -> ComputeOutput[1][1]/1(OutputB[x][y])
  Mux1/1 -> OutputI/1
  Mux/1 -> OutputH/1
  ComputeOutput[0][0]/1(OutputH[x][y]) -> Mux/1
  ComputeOutput[0][1]/1(OutputH[x][y]) -> Mux/2
  ComputeOutput[1][0]/1(OutputH[x][y]) -> Mux/3
  ComputeOutput[1][1]/1(OutputH[x][y]) -> Mux/4
  ComputeOutput[0][1]/2(OutputI[x][y]) -> Mux1/2
  ComputeOutput[0][0]/2(OutputI[x][y]) -> Mux1/1
  ComputeOutput[1][0]/2(OutputI[x][y]) -> Mux1/3
  ComputeOutput[1][1]/2(OutputI[x][y]) -> Mux1/4

== system Simulink_Model/Subsystem/Requirement7 ==
  note: Requirements implemented:
      | Requirement7
  OutputB : Inport
  SignalB : Inport  Port=2
  SignalC : Inport  Port=3
  ComputeOutputJ[0][0] : Subsystem
  ComputeOutputJ[0][1] : Subsystem
  ComputeOutputJ[1][0] : Subsystem
  ComputeOutputJ[1][1] : Subsystem
  Demux : Demux
  Demux1 : Demux
  Demux2 : Demux  Outputs=2
  Mux : Mux
  OutputJ : Outport
  wires:
  OutputB/1 -> Demux/1
  SignalB/1 -> Demux2/1
  SignalC/1 -> Demux1/1
  Demux/1 -> ComputeOutputJ[0][0]/1(OutputB[x][y])
  Demux/2 -> ComputeOutputJ[0][1]/1(OutputB[x][y])
  Demux/3 -> ComputeOutputJ[1][0]/1(OutputB[x][y])
  Demux/4 -> ComputeOutputJ[1][1]/1(OutputB[x][y])
  Demux2/1 -> ComputeOutputJ[0][1]/2(SignalB[x]), ComputeOutputJ[0][0]/2(SignalB[x])
  Demux2/2 -> ComputeOutputJ[1][1]/2(SignalB[x]), ComputeOutputJ[1][0]/2(SignalB[x])
  Demux1/1 -> ComputeOutputJ[0][0]/3(SignalC[x][y])
  Demux1/2 -> ComputeOutputJ[0][1]/3(SignalC[x][y])
  Demux1/3 -> ComputeOutputJ[1][0]/3(SignalC[x][y])
  Demux1/4 -> ComputeOutputJ[1][1]/3(SignalC[x][y])
  Mux/1 -> OutputJ/1
  ComputeOutputJ[0][0]/1(OutputJ[x][y]) -> Mux/1
  ComputeOutputJ[0][1]/1(OutputJ[x][y]) -> Mux/2
  ComputeOutputJ[1][0]/1(OutputJ[x][y]) -> Mux/3
  ComputeOutputJ[1][1]/1(OutputJ[x][y]) -> Mux/4

== system Simulink_Model/Subsystem/Requirement8 ==
  note: Requirements implemented:
      | Requirement8
  OutputB : Inport
  OutputJ : Inport  Port=2
  OutputKOld : Inport  Port=3
  OutputLOld : Inport  Port=4
  ComputeOutput[0][0] : Subsystem
  ComputeOutput[0][1] : Subsystem
  ComputeOutput[1][0] : Subsystem
  ComputeOutput[1][1] : Subsystem
  Demux{,1..3} (4 alike) : Demux
  Mux : Mux
  Mux1 : Mux
  OutputK : Outport
  OutputL : Outport  Port=2
  wires:
  OutputB/1 -> Demux/1
  OutputJ/1 -> Demux1/1
  OutputKOld/1 -> Demux2/1
  OutputLOld/1 -> Demux3/1
  Demux/1 -> ComputeOutput[0][0]/1(OutputB[x][y])
  Demux/2 -> ComputeOutput[0][1]/1(OutputB[x][y])
  Demux/3 -> ComputeOutput[1][0]/1(OutputB[x][y])
  Demux/4 -> ComputeOutput[1][1]/1(OutputB[x][y])
  Demux1/1 -> ComputeOutput[0][0]/2(OutputJ[x][y])
  Demux1/2 -> ComputeOutput[0][1]/2(OutputJ[x][y])
  Demux1/3 -> ComputeOutput[1][0]/2(OutputJ[x][y])
  Demux1/4 -> ComputeOutput[1][1]/2(OutputJ[x][y])
  Demux2/1 -> ComputeOutput[0][0]/3(OutputKOld[x][y])
  Demux2/2 -> ComputeOutput[0][1]/3(OutputKOld[x][y])
  Demux2/3 -> ComputeOutput[1][0]/3(OutputKOld[x][y])
  Demux2/4 -> ComputeOutput[1][1]/3(OutputKOld[x][y])
  Demux3/1 -> ComputeOutput[0][0]/4(OutputLOld[x][y])
  Demux3/2 -> ComputeOutput[0][1]/4(OutputLOld[x][y])
  Demux3/3 -> ComputeOutput[1][0]/4(OutputLOld[x][y])
  Demux3/4 -> ComputeOutput[1][1]/4(OutputLOld[x][y])
  Mux/1 -> OutputK/1
  Mux1/1 -> OutputL/1
  ComputeOutput[0][0]/1(OutputK[x][y]) -> Mux/1
  ComputeOutput[0][1]/1(OutputK[x][y]) -> Mux/2
  ComputeOutput[1][0]/1(OutputK[x][y]) -> Mux/3
  ComputeOutput[1][1]/1(OutputK[x][y]) -> Mux/4
  ComputeOutput[0][0]/2(OutputL[x][y]) -> Mux1/1
  ComputeOutput[0][1]/2(OutputL[x][y]) -> Mux1/2
  ComputeOutput[1][0]/2(OutputL[x][y]) -> Mux1/3
  ComputeOutput[1][1]/2(OutputL[x][y]) -> Mux1/4

== system Simulink_Model/Subsystem/Requirement9 ==
  note: Requirements implemented:
      | Requirement9
  OutputE : Inport
  ComputeOutputM[0] : Subsystem
  ComputeOutputM[0]1 : Subsystem
  Demux : Demux
  Mux : Mux  Inputs=2
  OutputM : Outport
  wires:
  Mux/1 -> OutputM/1
  ComputeOutputM[0]/1(OutputM[x]) -> Mux/1
  ComputeOutputM[0]1/1(OutputM[x]) -> Mux/2
  OutputE/1 -> Demux/1
  Demux/1 -> ComputeOutputM[0]/1(OutputE[x][0])
  Demux/2 -> ComputeOutputM[0]/2(OutputE[x][1])
  Demux/3 -> ComputeOutputM[0]1/1(OutputE[x][0])
  Demux/4 -> ComputeOutputM[0]1/2(OutputE[x][1])

== system Simulink_Model/Subsystem/Verification2 ==
  note: Requirements implemented:
      | Verification2
  OutputB : Inport
  ComputeStateB[0] : Subsystem
  ComputeStateB[1] : Subsystem
  Demux : Demux
  Mux : Mux  Inputs=2
  StateB : Outport
  wires:
  OutputB/1 -> Demux/1
  Mux/1 -> StateB/1
  Demux/1 -> ComputeStateB[0]/1(OutputB[x][0])
  Demux/2 -> ComputeStateB[0]/2(OutputB[x][1])
  Demux/3 -> ComputeStateB[1]/1(OutputB[x][0])
  Demux/4 -> ComputeStateB[1]/2(OutputB[x][1])
  ComputeStateB[0]/1(StateB[x]) -> Mux/1
  ComputeStateB[1]/1(StateB[x]) -> Mux/2

== system Simulink_Model/Subsystem/Verification3 ==
  note: Requirements implemented:
      | Verification3
  OutputY : Inport
  Constant : Constant  Value=0
  Constant1 : Constant  Value=2
  Demux : Demux  Outputs=2
  Product : Product
  Relational Operator : RelationalOperator  Operator=<  OutDataTypeStr=boolean  RndMeth=Simplest
  Subsystem Reference : Subsystem  ReferencedSubsystem=ComputeState
  Switch : Switch  Criteria=u2 > Threshold
  StateC : Outport
  wires:
  OutputY/1 -> Demux/1
  Demux/1 -> Product/1
  Demux/2 -> Product/2
  Product/1 -> Relational Operator/2
  Constant/1 -> Switch/1, Relational Operator/1
  Relational Operator/1 -> Switch/2
  Constant1/1 -> Switch/3
  Switch/1 -> Subsystem Reference/1
  Subsystem Reference/1 -> StateC/1

== system Simulink_Model/Subsystem/Verification4 ==
  note: Requirements implemented:
      | Verification4
  OutputP : Inport
  ComputeStateD[0] : Subsystem
  ComputeStateD[1] : Subsystem
  Demux : Demux  Outputs=2
  Mux : Mux  Inputs=2
  StateD : Outport
  wires:
  OutputP/1 -> Demux/1
  Demux/1 -> ComputeStateD[0]/1(OutputP[x])
  Demux/2 -> ComputeStateD[1]/1(OutputP[x])
  ComputeStateD[0]/1(StateD[X]) -> Mux/1
  ComputeStateD[1]/1(StateD[X]) -> Mux/2
  Mux/1 -> StateD/1

== system Simulink_Model/Subsystem/Verification5 ==
  note: Requirements implemented:
      | Verification5
  OutputP : Inport
  ComputeStateE[0] : Subsystem
  ComputeStateE[0]1 : Subsystem
  Demux : Demux  Outputs=2
  Mux : Mux  Inputs=2
  StateE : Outport
  wires:
  OutputP/1 -> Demux/1
  Mux/1 -> StateE/1
  Demux/1 -> ComputeStateE[0]1/2(OutputP[1]), ComputeStateE[0]/1(OutputP[0])
  Demux/2 -> ComputeStateE[0]/2(OutputP[1]), ComputeStateE[0]1/1(OutputP[0])
  ComputeStateE[0]/1(StateE[x]) -> Mux/1
  ComputeStateE[0]1/1(StateE[x]) -> Mux/2

== system Simulink_Model/Subsystem/Verification6 ==
  note: Requirements implemented:
      | Verification6
  StateE : Inport
  ComputeStateE[0] : Subsystem
  ComputeStateE[1] : Subsystem
  Demux : Demux  Outputs=2
  Mux : Mux  Inputs=2
  StateF : Outport
  wires:
  StateE/1 -> Demux/1
  Mux/1 -> StateF/1
  Demux/1 -> ComputeStateE[0]/1(StateE[x])
  ComputeStateE[0]/1(StateF[x]) -> Mux/1
  Demux/2 -> ComputeStateE[1]/1(StateE[x])
  ComputeStateE[1]/1(StateF[x]) -> Mux/2

== system Simulink_Model/Subsystem/Verification8 ==
  note: Requirements implemented:
      | Verification8
  OutputAB : Inport
  Abs : Abs
  Constant : Constant  Value=2
  Constant1 : Constant  Value=0
  Constant3 : Constant  Value=ConstantO
  Demux : Demux  Outputs=2
  Relational Operator : RelationalOperator  Operator=>  OutDataTypeStr=boolean  RndMeth=Simplest
  Subsystem Reference : Subsystem  ReferencedSubsystem=ComputeState
  Sum : Sum  Inputs=|+-
  Switch : Switch  Criteria=u2 > Threshold
  StateG : Outport
  wires:
  OutputAB/1 -> Demux/1
  Demux/1 -> Sum/1
  Demux/2 -> Sum/2
  Sum/1 -> Abs/1
  Abs/1 -> Relational Operator/1
  Constant3/1 -> Relational Operator/2  "ConstantO"
  Relational Operator/1 -> Switch/2
  Constant1/1 -> Switch/3
  Constant/1 -> Switch/1
  Switch/1 -> Subsystem Reference/1
  Subsystem Reference/1 -> StateG/1

== system Simulink_Model/Subsystem/Requirement12/ComputeOutput0 ==
  OutputM[x] : Inport
  OutputPOld[x] : Inport  Port=2
  OutputQOld[x] : Inport  Port=3
  Constant1 : Constant  Value=ConstantC
  Constant4 : Constant  Value=ConstantD
  Delay : Delay  DelayLength=1  InitialCondition=0
  Delay1 : Delay  DelayLength=1  InitialCondition=0
  Divide : Product  Inputs=*/
  Product : Product
  Product1 : Product
  Product2 : Product
  Subtract : Sum  Inputs=+-
  Sum : Sum  Inputs=|+++
  Sum1 : Sum  Inputs=|++
  OutputP[x] : Outport
  OutputQ[x] : Outport  Port=2
  wires:
  OutputPOld[x]/1 -> Delay/1
  Constant4/1 -> Sum1/2, Product/2  "ConstantD"
  Constant1/1 -> Sum1/1, Product1/1  "ConstantC"
  OutputM[x]/1 -> Product1/2
  Product1/1 -> Sum/1
  Product/1 -> Sum/2
  OutputQOld[x]/1 -> Delay1/1
  Sum/1 -> Subtract/1, Divide/1
  Sum1/1 -> Product2/2, Divide/2
  Divide/1 -> Product2/1, OutputP[x]/1
  Product2/1 -> Subtract/2
  Subtract/1 -> OutputQ[x]/1
  Delay/1 -> Product/1
  Delay1/1 -> Sum/3

== system Simulink_Model/Subsystem/Requirement12/ComputeOutput1 ==
  OutputM[x] : Inport
  OutputPOld[x] : Inport  Port=2
  OutputQOld[x] : Inport  Port=3
  Constant1 : Constant  Value=ConstantC
  Constant4 : Constant  Value=ConstantD
  Delay : Delay  DelayLength=1  InitialCondition=0
  Delay1 : Delay  DelayLength=1  InitialCondition=0
  Divide : Product  Inputs=*/
  Product : Product
  Product1 : Product
  Product2 : Product
  Subtract : Sum  Inputs=+-
  Sum : Sum  Inputs=|+++
  Sum1 : Sum  Inputs=|++
  OutputP[x] : Outport
  OutputQ[x] : Outport  Port=2
  wires:
  OutputPOld[x]/1 -> Delay/1
  Constant4/1 -> Sum1/2, Product/2  "ConstantD"
  Constant1/1 -> Sum1/1, Product1/1  "ConstantC"
  OutputM[x]/1 -> Product1/2
  Product1/1 -> Sum/1
  Product/1 -> Sum/2
  OutputQOld[x]/1 -> Delay1/1
  Sum/1 -> Subtract/1, Divide/1
  Sum1/1 -> Product2/2, Divide/2
  Divide/1 -> Product2/1, OutputP[x]/1
  Product2/1 -> Subtract/2
  Subtract/1 -> OutputQ[x]/1
  Delay/1 -> Product/1
  Delay1/1 -> Sum/3

== system Simulink_Model/Subsystem/Requirement14/ComputeOutput0 ==
  OutputN[x] : Inport
  OutputROld[x] : Inport  Port=2
  OutputSOld[x] : Inport  Port=3
  Constant1 : Constant  Value=ConstantC
  Constant2 : Constant  Value=ConstantD
  Delay1 : Delay  DelayLength=1  InitialCondition=0
  Delay2 : Delay  DelayLength=1  InitialCondition=0
  Divide : Product  Inputs=*/  RndMeth=Nearest
  Product : Product
  Product1 : Product
  Product2 : Product
  Subtract : Sum  Inputs=+-
  Sum : Sum  Inputs=|+++
  Sum1 : Sum  Inputs=|++
  OutputR[x] : Outport
  OutputS[x] : Outport  Port=2
  wires:
  Constant2/1 -> Product/2, Sum1/2  "ConstantD"
  Constant1/1 -> Sum1/1, Product1/1  "ConstantC"
  OutputN[x]/1 -> Product1/2
  Product1/1 -> Sum/1
  OutputSOld[x]/1 -> Delay1/1
  Sum/1 -> Subtract/1, Divide/1
  Sum1/1 -> Product2/2, Divide/2
  Product2/1 -> Subtract/2
  Subtract/1 -> OutputS[x]/1
  Delay1/1 -> Sum/3
  Product/1 -> Sum/2
  Divide/1 -> Product2/1, OutputR[x]/1
  OutputROld[x]/1 -> Delay2/1
  Delay2/1 -> Product/1

== system Simulink_Model/Subsystem/Requirement14/ComputeOutput1 ==
  OutputN[x] : Inport
  OutputROld[x] : Inport  Port=2
  OutputSOld[x] : Inport  Port=3
  Constant1 : Constant  Value=ConstantC
  Constant2 : Constant  Value=ConstantD
  Delay : Delay  DelayLength=1  InitialCondition=0
  Delay1 : Delay  DelayLength=1  InitialCondition=0
  Divide : Product  Inputs=*/
  Product : Product
  Product1 : Product
  Product2 : Product
  Subtract : Sum  Inputs=+-
  Sum : Sum  Inputs=|+++
  Sum1 : Sum  Inputs=|++
  OutputR[x] : Outport
  OutputS[x] : Outport  Port=2
  wires:
  OutputROld[x]/1 -> Delay/1
  Constant2/1 -> Product/2, Sum1/2  "ConstantD"
  Constant1/1 -> Sum1/1, Product1/1  "ConstantC"
  OutputN[x]/1 -> Product1/2
  Product1/1 -> Sum/1
  Product/1 -> Sum/2
  OutputSOld[x]/1 -> Delay1/1
  Sum/1 -> Subtract/1, Divide/1
  Sum1/1 -> Product2/2, Divide/2
  Divide/1 -> Product2/1, OutputR[x]/1
  Product2/1 -> Subtract/2
  Subtract/1 -> OutputS[x]/1
  Delay/1 -> Product/1
  Delay1/1 -> Sum/3

== system Simulink_Model/Subsystem/Requirement15/ComputeOutput0 ==
  OutputO[x] : Inport
  OutputTOld[x] : Inport  Port=2
  OutputUOld[x] : Inport  Port=3
  Constant1 : Constant  Value=ConstantC
  Constant4 : Constant  Value=ConstantD
  Delay : Delay  DelayLength=1  InitialCondition=0
  Delay1 : Delay  DelayLength=1  InitialCondition=0
  Divide : Product  Inputs=*/
  Product : Product
  Product1 : Product
  Product2 : Product
  Subtract : Sum  Inputs=+-
  Sum : Sum  Inputs=|+++
  Sum1 : Sum  Inputs=|++
  OutputT[x] : Outport
  OutputU[x] : Outport  Port=2
  wires:
  OutputTOld[x]/1 -> Delay/1
  Constant4/1 -> Sum1/2, Product/2  "ConstantD"
  Constant1/1 -> Sum1/1, Product1/1  "ConstantC"
  OutputO[x]/1 -> Product1/2
  Product1/1 -> Sum/1
  Product/1 -> Sum/2
  OutputUOld[x]/1 -> Delay1/1
  Sum/1 -> Subtract/1, Divide/1
  Sum1/1 -> Product2/2, Divide/2
  Divide/1 -> Product2/1, OutputT[x]/1
  Product2/1 -> Subtract/2
  Subtract/1 -> OutputU[x]/1
  Delay/1 -> Product/1
  Delay1/1 -> Sum/3

== system Simulink_Model/Subsystem/Requirement15/ComputeOutput1 ==
  OutputO[x] : Inport
  OutputTOld[x] : Inport  Port=2
  OutputUOld[x] : Inport  Port=3
  Constant1 : Constant  Value=ConstantC
  Constant4 : Constant  Value=ConstantD
  Delay : Delay  DelayLength=1  InitialCondition=0
  Delay1 : Delay  DelayLength=1  InitialCondition=0
  Divide : Product  Inputs=*/
  Product : Product
  Product1 : Product
  Product2 : Product
  Subtract : Sum  Inputs=+-
  Sum : Sum  Inputs=|+++
  Sum1 : Sum  Inputs=|++
  OutputT[x] : Outport
  OutputU[x] : Outport  Port=2
  wires:
  OutputTOld[x]/1 -> Delay/1
  Constant4/1 -> Sum1/2, Product/2  "ConstantD"
  Constant1/1 -> Sum1/1, Product1/1  "ConstantC"
  OutputO[x]/1 -> Product1/2
  Product1/1 -> Sum/1
  Product/1 -> Sum/2
  OutputUOld[x]/1 -> Delay1/1
  Sum/1 -> Subtract/1, Divide/1
  Sum1/1 -> Product2/2, Divide/2
  Divide/1 -> Product2/1, OutputT[x]/1
  Product2/1 -> Subtract/2
  Subtract/1 -> OutputU[x]/1
  Delay/1 -> Product/1
  Delay1/1 -> Sum/3

== system Simulink_Model/Subsystem/Requirement23/OutputX[0][0] ==
  OutputE[x][y] : Inport
  OutputEOld[x][y] : Inport  Port=2
  Abs : Abs
  Abs1 : Abs
  Constant : Constant  Value=200000
  Constant1 : Constant  Value=2
  Constant4 : Constant  Value=ConstantF
  Divide : Product  Inputs=*/
  Product : Product
  Product1 : Product
  Sum : Sum  Inputs=|+-
  Sum1 : Sum  Inputs=|++
  OutputX[x][y] : Outport
  wires:
  OutputE[x][y]/1 -> Abs/1
  OutputEOld[x][y]/1 -> Abs1/1
  Abs1/1 -> Sum/2
  Abs/1 -> Sum/1
  Sum/1 -> Product/2
  Constant/1 -> Product/1
  Product/1 -> Sum1/1
  Constant4/1 -> Sum1/2, Product1/1  "ConstantF"
  Constant1/1 -> Product1/2
  Sum1/1 -> Divide/1
  Product1/1 -> Divide/2
  Divide/1 -> OutputX[x][y]/1

== system Simulink_Model/Subsystem/Requirement23/OutputX[0][1] ==
  OutputE[x][y] : Inport
  OutputEOld[x][y] : Inport  Port=2
  Abs : Abs
  Abs1 : Abs
  Constant : Constant  Value=200000
  Constant1 : Constant  Value=2
  Constant4 : Constant  Value=ConstantF
  Divide : Product  Inputs=*/
  Product : Product
  Product1 : Product
  Sum : Sum  Inputs=|+-
  Sum1 : Sum  Inputs=|++
  OutputX[x][y] : Outport
  wires:
  OutputE[x][y]/1 -> Abs/1
  OutputEOld[x][y]/1 -> Abs1/1
  Abs1/1 -> Sum/2
  Abs/1 -> Sum/1
  Sum/1 -> Product/2
  Constant/1 -> Product/1
  Product/1 -> Sum1/1
  Constant4/1 -> Sum1/2, Product1/1  "ConstantF"
  Constant1/1 -> Product1/2
  Sum1/1 -> Divide/1
  Product1/1 -> Divide/2
  Divide/1 -> OutputX[x][y]/1

== system Simulink_Model/Subsystem/Requirement23/OutputX[1][0] ==
  OutputE[x][y] : Inport
  OutputEOld[x][y] : Inport  Port=2
  Abs : Abs
  Abs1 : Abs
  Constant : Constant  Value=200000
  Constant1 : Constant  Value=2
  Constant4 : Constant  Value=ConstantF
  Divide : Product  Inputs=*/
  Product : Product
  Product1 : Product
  Sum : Sum  Inputs=|+-
  Sum1 : Sum  Inputs=|++
  OutputX[x][y] : Outport
  wires:
  OutputE[x][y]/1 -> Abs/1
  OutputEOld[x][y]/1 -> Abs1/1
  Abs1/1 -> Sum/2
  Abs/1 -> Sum/1
  Sum/1 -> Product/2
  Constant/1 -> Product/1
  Product/1 -> Sum1/1
  Constant4/1 -> Sum1/2, Product1/1  "ConstantF"
  Constant1/1 -> Product1/2
  Sum1/1 -> Divide/1
  Product1/1 -> Divide/2
  Divide/1 -> OutputX[x][y]/1

== system Simulink_Model/Subsystem/Requirement23/OutputX[1][1] ==
  OutputE[x][y] : Inport
  OutputEOld[x][y] : Inport  Port=2
  Abs : Abs
  Abs1 : Abs
  Constant : Constant  Value=200000
  Constant1 : Constant  Value=2
  Constant4 : Constant  Value=ConstantF
  Divide : Product  Inputs=*/
  Product : Product
  Product1 : Product
  Sum : Sum  Inputs=|+-
  Sum1 : Sum  Inputs=|++
  OutputX[x][y] : Outport
  wires:
  OutputE[x][y]/1 -> Abs/1
  OutputEOld[x][y]/1 -> Abs1/1
  Abs1/1 -> Sum/2
  Abs/1 -> Sum/1
  Sum/1 -> Product/2
  Constant/1 -> Product/1
  Product/1 -> Sum1/1
  Constant4/1 -> Sum1/2, Product1/1  "ConstantF"
  Constant1/1 -> Product1/2
  Sum1/1 -> Divide/1
  Product1/1 -> Divide/2
  Divide/1 -> OutputX[x][y]/1

== system Simulink_Model/Subsystem/Requirement24/OutputY[0] ==
  OutputX[x][0] : Inport
  OutputX[x][1] : Inport  Port=2
  Constant : Constant
  Constant1 : Constant  Value=2
  Divide : Product  Inputs=*/
  Sum : Sum  Inputs=|+++
  OutputY[x] : Outport
  wires:
  Constant/1 -> Sum/1
  OutputX[x][0]/1 -> Sum/2
  OutputX[x][1]/1 -> Sum/3
  Sum/1 -> Divide/1
  Constant1/1 -> Divide/2
  Divide/1 -> OutputY[x]/1

== system Simulink_Model/Subsystem/Requirement24/OutputY[1] ==
  OutputX[x][0] : Inport
  OutputX[x][1] : Inport  Port=2
  Constant : Constant
  Constant1 : Constant  Value=2
  Divide : Product  Inputs=*/
  Sum : Sum  Inputs=|+++
  OutputY[x] : Outport
  wires:
  Constant/1 -> Sum/1
  OutputX[x][0]/1 -> Sum/2
  OutputX[x][1]/1 -> Sum/3
  Sum/1 -> Divide/1
  Constant1/1 -> Divide/2
  Divide/1 -> OutputY[x]/1

== system Simulink_Model/Subsystem/Requirement25/Subsystem ==
  OutputB[x][0] : Inport
  OutputC[x] : Inport  Port=2
  OutputAAOld[x] : Inport  Port=3
  Constant1 : Constant  Value=ConstantG
  Constant2 : Constant  Value=ConstantB
  Constant3 : Constant  Value=ConstantH
  Constant4 : Constant  Value=ConstantC
  Divide : Product  Inputs=*/
  Plus : Sum
  Product : Product  Inputs=4
  Product1 : Product
  Product2 : Product
  Sum : Sum  Inputs=|-+
  OutputZ[x] : Outport
  OutputAA[x] : Outport  Port=2
  wires:
  Constant1/1 -> Product/1  "ConstantG"
  Constant2/1 -> Product/2  "ConstantB"
  OutputB[x][0]/1 -> Product/3
  OutputC[x]/1 -> Product/4
  Product/1 -> Plus/1
  OutputAAOld[x]/1 -> Plus/2
  Constant3/1 -> Product1/1  "ConstantH"
  Constant4/1 -> Product1/2  "ConstantC"
  Plus/1 -> Sum/2, Divide/1
  Product1/1 -> Product2/2, Divide/2
  Divide/1 -> Product2/1, OutputZ[x]/1
  Sum/1 -> OutputAA[x]/1
  Product2/1 -> Sum/1

== system Simulink_Model/Subsystem/Requirement25/Subsystem1 ==
  OutputB[x][0] : Inport
  OutputC[x] : Inport  Port=2
  OutputAAOld[x] : Inport  Port=3
  Constant1 : Constant  Value=ConstantG
  Constant2 : Constant  Value=ConstantB
  Constant3 : Constant  Value=ConstantH
  Constant4 : Constant  Value=ConstantC
  Divide : Product  Inputs=*/
  Plus : Sum
  Product : Product  Inputs=4
  Product1 : Product
  Product2 : Product
  Sum : Sum  Inputs=|-+
  OutputZ[x] : Outport
  OutputAA[x] : Outport  Port=2
  wires:
  Constant1/1 -> Product/1  "ConstantG"
  Constant2/1 -> Product/2  "ConstantB"
  OutputB[x][0]/1 -> Product/3
  OutputC[x]/1 -> Product/4
  Product/1 -> Plus/1
  OutputAAOld[x]/1 -> Plus/2
  Constant3/1 -> Product1/1  "ConstantH"
  Constant4/1 -> Product1/2  "ConstantC"
  Plus/1 -> Sum/2, Divide/1
  Product1/1 -> Product2/2, Divide/2
  Divide/1 -> Product2/1, OutputZ[x]/1
  Sum/1 -> OutputAA[x]/1
  Product2/1 -> Sum/1

== system Simulink_Model/Subsystem/Requirement26/Subsystem ==
  OutputZ[x] : Inport
  OutputABOld[x] : Inport  Port=2
  Sum : Sum  Inputs=|++
  OutputAB[x] : Outport
  wires:
  OutputZ[x]/1 -> Sum/1
  OutputABOld[x]/1 -> Sum/2
  Sum/1 -> OutputAB[x]/1

== system Simulink_Model/Subsystem/Requirement26/Subsystem1 ==
  OutputZ[x] : Inport
  OutputABOld[x] : Inport  Port=2
  Sum : Sum  Inputs=|++
  OutputAB[x] : Outport
  wires:
  OutputZ[x]/1 -> Sum/1
  OutputABOld[x]/1 -> Sum/2
  Sum/1 -> OutputAB[x]/1
